simulink model "mass_spring_system_model"  (Simulink 7.7)
settings: Solver=ode45  StartTime=0.0  StopTime=T_end  RelTol=1e-3
undefined symbols (not defined in the file): c_id, d_id, m_id, Td
settings Model: Creator=Rumetshofer  LastModifiedBy=Rumetshofer

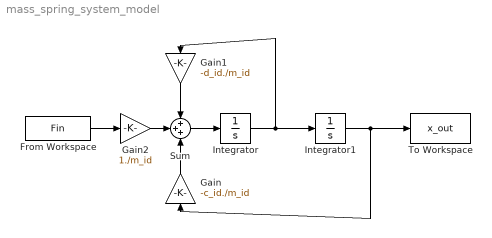
== system mass_spring_system_model ==
  From Workspace : FromWorkspace  VariableName=Fin  SampleTime=Td
  Gain : Gain  Gain=-c_id./m_id
  Gain1 : Gain  Gain=-d_id./m_id
  Gain2 : Gain  Gain=1./m_id
  Integrator : Integrator
  Integrator1 : Integrator
  Sum : Sum  Inputs=+++
  To Workspace : ToWorkspace  VariableName=x_out  SampleTime=Td  SaveFormat=Array
  wires:
  Integrator1/1 -> To Workspace/1, Gain/1
  Integrator/1 -> Integrator1/1, Gain1/1
  Sum/1 -> Integrator/1
  Gain/1 -> Sum/3
  Gain1/1 -> Sum/1
  From Workspace/1 -> Gain2/1
  Gain2/1 -> Sum/2
